simulink model "StartEinerZweistufigenRakete"  (R2014b)
settings: Solver=ode45  StartTime=0.0  StopTime=600  RelTol=1e-3
settings Model: Creator=Florian  LastModifiedBy=Florian

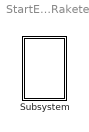
== system StartEinerZweistufigenRakete ==
  Subsystem : Subsystem  mask{m1_leer=500, m2_leer=1000, St1_Treibstoff=4000, St2_Treibstoff=1500, Durchsatz_1=20, Durchsatz_2=15, SchubProDurchsatz=4000}
      mask prompts: SchubProDurchsatz "SchubProDurchsatz  [N/(kg/s)]"

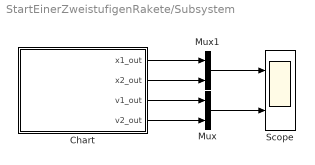
== system StartEinerZweistufigenRakete/Subsystem ==
  Chart : Stateflow chart  TreatAsAtomicUnit=on
  Mux : Mux  Inputs=2
  Mux1 : Mux  Inputs=2
  Scope : Scope  NumInputPorts=2
      settings: TimeRange=600  YMin=-200000~-3000  YMax=1400000~5000  Decimation=2
  wires:
  Mux/1 -> Scope/2
  Mux1/1 -> Scope/1
  Chart/1(x1_out) -> Mux1/1
  Chart/2(x2_out) -> Mux1/2
  Chart/4(v2_out) -> Mux/2
  Chart/3(v1_out) -> Mux/1

== stateflow chart StartEinerZweistufigenRakete/Subsystem/Chart ==
  settings: updateMethod=CONTINUOUS
  state StuffenGemeinsam
    during:
    %Derivatives
    [v1_dot, v2_dot] = Acc1();
    x1_dot = v1;
    x2_dot = v2;
    m1_dot = -Durchsatz_1;
    m2_dot = 0;
    %Output
    x1_out = x1;
    x2_out = x2;
    v1_out = v1;
    v2_out = v2;
  state StuffenGetrennt
    during:
    %Derivatives
    [v1_dot, v2_dot] = Acc2();
    x1_dot = v1;
    x2_dot = v2;
    m1_dot = 0;
    m2_dot = -Durchsatz_2;
    %Output
    x1_out = x1;
    x2_out = x2;
    v1_out = v1;
    v2_out = v2;
  state Stuffe2Ausgebrannt
    during:
    %Derivatives
    [v1_dot, v2_dot] = Acc3();
    x1_dot = v1;
    x2_dot = v2;
    m1_dot = 0;
    m2_dot = 0;
    %Output
    x1_out = x1;
    x2_out = x2;
    v1_out = v1;
    v2_out = v2;
  StuffenGetrennt -> Stuffe2Ausgebrannt : [m2 <= m2_leer]
  StuffenGemeinsam -> StuffenGetrennt : [m1 <= m1_leer]
  (default) -> StuffenGemeinsam : {init();}
  data: a1 function_output double; a2 function_output double; a1 function_output double; a2 function_output double; a1 function_output double; a2 function_output double; m1_leer parameter; St1_Treibstoff parameter; Durchsatz_1 parameter; m2_leer parameter; St2_Treibstoff parameter; Durchsatz_2 parameter; SchubProDurchsatz parameter; Erdmasse constant double size=1 =5.9736*10^24; Erdradius constant double size=1 =6378000; Gravitation constant double size=1 =66.743*10^-12; v1 local; x1 local; v2 local; x2 local; m1 local; m2 local; x1_out output; x2_out output; v1_out output; v2_out output
  data v1 settings: updateMethod=SF_CONTINUOUS_TIME_DATA
  data x1 settings: updateMethod=SF_CONTINUOUS_TIME_DATA
  data v2 settings: updateMethod=SF_CONTINUOUS_TIME_DATA
  data x2 settings: updateMethod=SF_CONTINUOUS_TIME_DATA
  data m1 settings: updateMethod=SF_CONTINUOUS_TIME_DATA
  data m2 settings: updateMethod=SF_CONTINUOUS_TIME_DATA
  function [a1,a2] = Acc1:
    | function [a1,a2] = Acc1 %Stufe 1 beschleunigt; Stufe 2 fliegt mit
    | 
    | MasseRakete = m1+m2;
    | 
    | FSchub  = SchubProDurchsatz*Durchsatz_1;
    | Fs      = Gravitation*(Erdmasse*MasseRakete)/((x1+Erdradius)^2);
    | 
    | a1      = (FSchub-Fs)/MasseRakete;
    | a2      = a1;
  function [a1,a2] = Acc3:
    | function [a1,a2] = Acc3 % Beide Stufen leer
    | 
    | FsStufe1 = Gravitation*(Erdmasse*m1)/((x1+Erdradius)^2); 
    | FsStufe2 = Gravitation*(Erdmasse*m2)/((x2+Erdradius)^2); 
    |  
    | a1       = -FsStufe1/m1; 
    | a2       = -FsStufe2/m2;
  function [a1,a2] = Acc2:
    | function [a1,a2] = Acc2 %Stufe 1 wird abgetrennt; Stufe2 beschleunigt
    | 
    | 
    | FsStufe1 = Gravitation*(Erdmasse*m1)/((x1+Erdradius)^2); %Gravitationskraft Stufe1
    | FsStufe2 = Gravitation*(Erdmasse*m2)/((x2+Erdradius)^2); %Gravitationskraft Stufe2
    | 
    | FSchub   = SchubProDurchsatz*Durchsatz_2; %Schubkraft
    | 
    | a1       = -FsStufe1/m1; 
    | a2       = (FSchub-FsStufe2)/m2;
  function init:
    | function init
    | %Beim Start = Auf der Erde & keine Geschwindigkeit
    | 
    | %Stufe 1
    | x1=0; 
    | v1=0;
    | 
    | %Stufe 2
    | x2=0;
    | v2=0;
    | 
    | m1=m1_leer+St1_Treibstoff;
    | m2=m2_leer+St2_Treibstoff;
